simulink model "bh_3d_pend_COMPONENT_MODEL"  (R2021b)
settings: Solver=ode45  StartTime=0.0  StopTime=10.0  RelTol=1e-5
undefined symbols (not defined in the file or in its folder): g, Lx, Ly, Lz, M_cart, m_pend, q0, q0_dot
settings Model: Creator=bhorton  LastModifiedBy=bhorton
settings SolverCC: ZeroCrossAlgorithm=Adaptive  AlgebraicLoopSolver=TrustRegion
settings DataIOCC: ReturnWorkspaceOutputs=off
settings DebuggingCC: SFMachineParentedDataDiag=warning  ArithmeticOperatorsInVariantConditions=warning
settings SFSimCC: SimUseLocalCustomCode=off  CustomCodeUndefinedFunction=UseInterfaceOnly
settings RTWCC: RTWUseLocalCustomCode=off
settings CodeAppCC: StateflowObjectComments=on

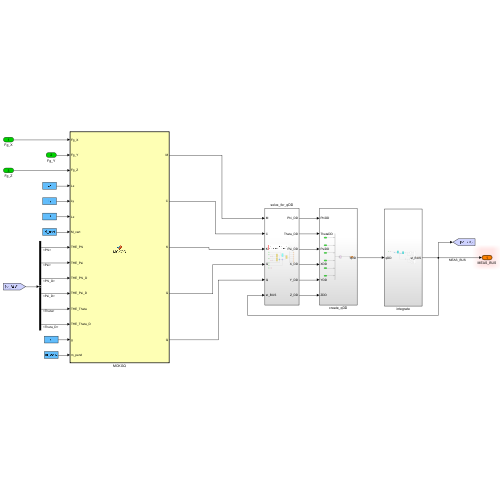
[thumbnail: Simulink's stored preview of the top-level diagram]
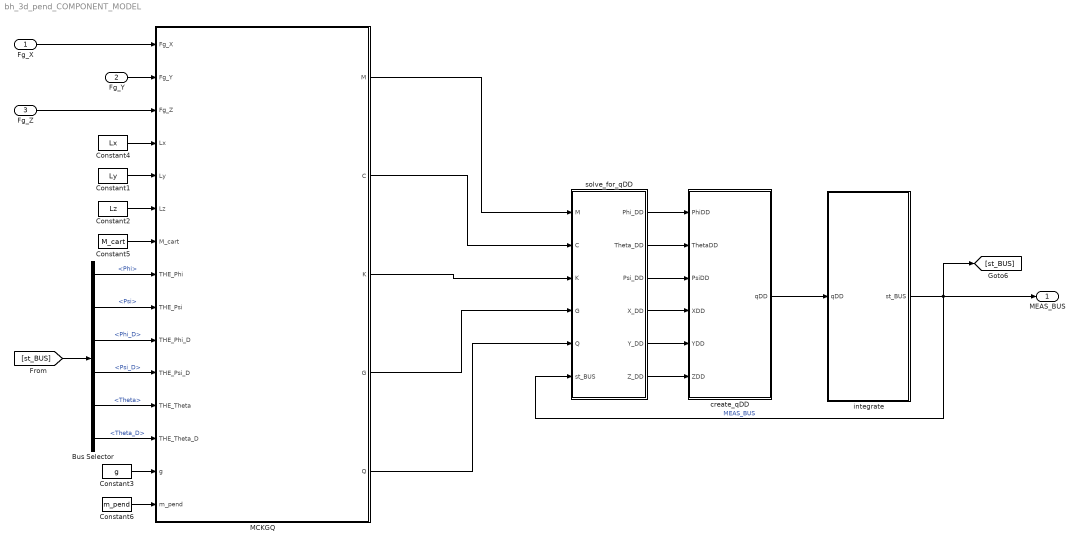
== system bh_3d_pend_COMPONENT_MODEL ==
  Fg_X : Inport
  Fg_Y : Inport  Port=2
  Fg_Z : Inport  Port=3
  Bus Selector : BusSelector  OutputSignals=Pos_list.Phi,Pos_list.Psi,Vel_list.Phi_D,Vel_list.Psi_D,Pos_list.Theta,Vel_list.Theta_D
  Constant1 : Constant  Value=Ly  OutDataTypeStr=Inherit: Inherit via back propagation
  Constant2 : Constant  Value=Lz  OutDataTypeStr=Inherit: Inherit via back propagation
  Constant3 : Constant  Value=g  OutDataTypeStr=Inherit: Inherit via back propagation
  Constant4 : Constant  Value=Lx  OutDataTypeStr=Inherit: Inherit via back propagation
  Constant5 : Constant  Value=M_cart  OutDataTypeStr=Inherit: Inherit via back propagation
  Constant6 : Constant  Value=m_pend  OutDataTypeStr=Inherit: Inherit via back propagation
  MCKGQ : MATLAB Function  TreatAsAtomicUnit=on
  create_qDD : Subsystem
  integrate : Subsystem
  solve_for_qDD : Subsystem
  MEAS_BUS : Outport  OutDataTypeStr=Bus: MEAS_BUS_SL_3D_PEND  VectorParamsAs1DForOutWhenUnconnected=off
  wires:
  solve_for_qDD/5(Y_DD) -> create_qDD/5(YDD)
  solve_for_qDD/3(Psi_DD) -> create_qDD/3(PsiDD)
  solve_for_qDD/2(Theta_DD) -> create_qDD/2(ThetaDD)
  integrate/1(st_BUS) -> MEAS_BUS/1, solve_for_qDD/6(st_BUS), [st_BUS]  "MEAS_BUS"
  solve_for_qDD/1(Phi_DD) -> create_qDD/1(PhiDD)
  solve_for_qDD/4(X_DD) -> create_qDD/4(XDD)
  solve_for_qDD/6(Z_DD) -> create_qDD/6(ZDD)
  MCKGQ/1(M) -> solve_for_qDD/1(M)
  MCKGQ/2(C) -> solve_for_qDD/2(C)
  MCKGQ/3(K) -> solve_for_qDD/3(K)
  MCKGQ/4(G) -> solve_for_qDD/4(G)
  MCKGQ/5(Q) -> solve_for_qDD/5(Q)
  create_qDD/1(qDD) -> integrate/1(qDD)
  Fg_Y/1 -> MCKGQ/2(Fg_Y)
  Fg_X/1 -> MCKGQ/1(Fg_X)
  Fg_Z/1 -> MCKGQ/3(Fg_Z)
  Constant5/1 -> MCKGQ/7(M_cart)
  Constant2/1 -> MCKGQ/6(Lz)
  Constant1/1 -> MCKGQ/5(Ly)
  Constant4/1 -> MCKGQ/4(Lx)
  Constant3/1 -> MCKGQ/14(g)
  Constant6/1 -> MCKGQ/15(m_pend)
  [st_BUS] -> Bus Selector/1
  Bus Selector/1 -> MCKGQ/8(THE_Phi)  "<Phi>"
  Bus Selector/2 -> MCKGQ/9(THE_Psi)  "<Psi>"
  Bus Selector/6 -> MCKGQ/13(THE_Theta_D)  "<Theta_D>"
  Bus Selector/5 -> MCKGQ/12(THE_Theta)  "<Theta>"
  Bus Selector/4 -> MCKGQ/11(THE_Psi_D)  "<Psi_D>"
  Bus Selector/3 -> MCKGQ/10(THE_Phi_D)  "<Phi_D>"

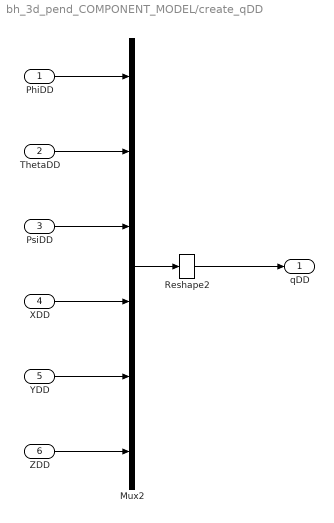
== system bh_3d_pend_COMPONENT_MODEL/create_qDD ==
  PhiDD : Inport
  ThetaDD : Inport  Port=2
  PsiDD : Inport  Port=3
  XDD : Inport  Port=4
  YDD : Inport  Port=5
  ZDD : Inport  Port=6
  Mux2 : Mux  Inputs=6
  Reshape2 : Reshape  OutputDimensionality=Column vector (2-D)
  qDD : Outport  VectorParamsAs1DForOutWhenUnconnected=off
  wires:
  PhiDD/1 -> Mux2/1
  ThetaDD/1 -> Mux2/2
  PsiDD/1 -> Mux2/3
  XDD/1 -> Mux2/4
  YDD/1 -> Mux2/5
  ZDD/1 -> Mux2/6
  Reshape2/1 -> qDD/1
  Mux2/1 -> Reshape2/1

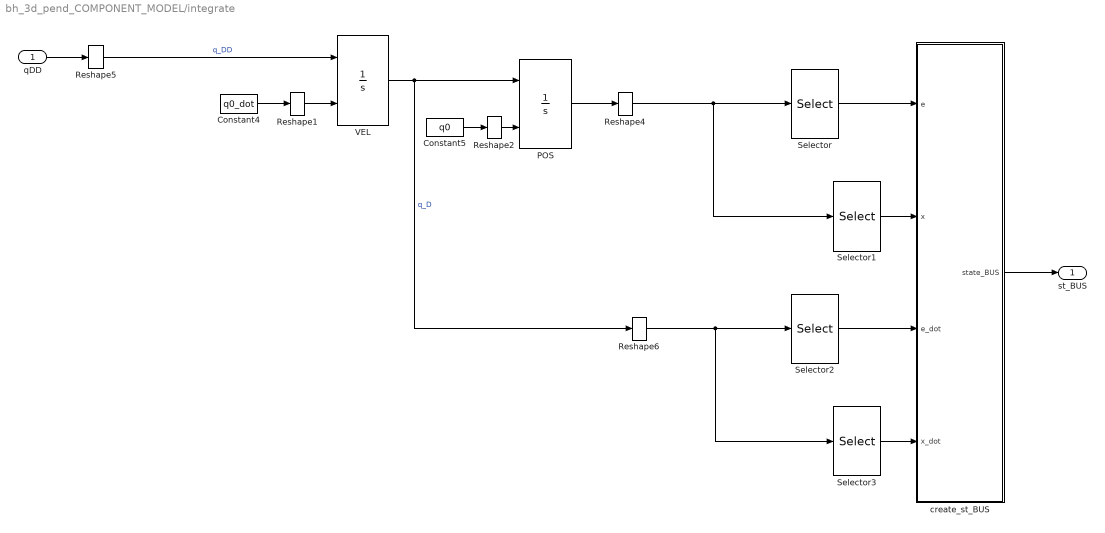
== system bh_3d_pend_COMPONENT_MODEL/integrate ==
  qDD : Inport
  Constant4 : Constant  Value=q0_dot  OutDataTypeStr=Inherit: Inherit via back propagation
  Constant5 : Constant  Value=q0  OutDataTypeStr=Inherit: Inherit via back propagation
  POS : Integrator  InitialConditionSource=external  ContinuousStateAttributes={'Phi', 'Theta', 'Psi', 'X','Y','Z'}
      settings: AttributesFormatString=%<ContinuousStateAttributes>
  Reshape{1..2,4..6} (5 alike) : Reshape  OutputDimensionality=Column vector (2-D)
  Selector : Selector  InputPortWidth=6  IndexOptions=Index vector (dialog)  Indices=1:3  OutputSizes=1
  Selector1 : Selector  InputPortWidth=6  IndexOptions=Index vector (dialog)  Indices=4:6  OutputSizes=1
  Selector2 : Selector  InputPortWidth=6  IndexOptions=Index vector (dialog)  Indices=1:3  OutputSizes=1
  Selector3 : Selector  InputPortWidth=6  IndexOptions=Index vector (dialog)  Indices=4:6  OutputSizes=1
  VEL : Integrator  InitialConditionSource=external  ContinuousStateAttributes={'Phi_D', 'Theta_D', 'Psi_D', 'X_D','Y_D','Z_D'}
      settings: AttributesFormatString=%<ContinuousStateAttributes>
  create_st_BUS : Subsystem
  st_BUS : Outport  VectorParamsAs1DForOutWhenUnconnected=off
  wires:
  qDD/1 -> Reshape5/1
  VEL/1 -> Reshape6/1, POS/1  "q_D"
  Reshape5/1 -> VEL/1  "q_DD"
  Constant5/1 -> Reshape2/1
  Constant4/1 -> Reshape1/1
  POS/1 -> Reshape4/1
  Reshape4/1 -> Selector1/1, Selector/1
  create_st_BUS/1(state_BUS) -> st_BUS/1
  Reshape1/1 -> VEL/2
  Reshape2/1 -> POS/2
  Selector3/1 -> create_st_BUS/4(x_dot)
  Selector2/1 -> create_st_BUS/3(e_dot)
  Selector1/1 -> create_st_BUS/2(x)
  Selector/1 -> create_st_BUS/1(e)
  Reshape6/1 -> Selector3/1, Selector2/1

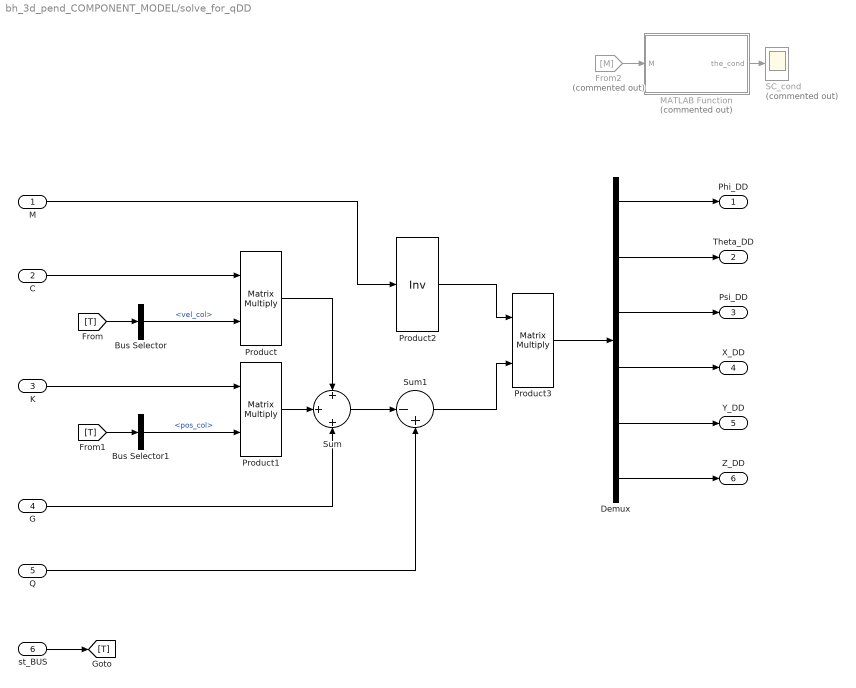
== system bh_3d_pend_COMPONENT_MODEL/solve_for_qDD ==
  M : Inport
  C : Inport  Port=2
  K : Inport  Port=3
  G : Inport  Port=4
  Q : Inport  Port=5
  st_BUS : Inport  Port=6
  Bus Selector : BusSelector  OutputSignals=vel_col
  Bus Selector1 : BusSelector  OutputSignals=pos_col
  Demux : Demux  Outputs=6
  From2 : From  Commented=on  GotoTag=M
  MATLAB Function : MATLAB Function  Commented=on  TreatAsAtomicUnit=on
  Product : Product  Multiplication=Matrix(*)
  Product1 : Product  Multiplication=Matrix(*)
  Product2 : Product  Inputs=/  Multiplication=Matrix(*)
  Product3 : Product  Multiplication=Matrix(*)
  SC_cond : Scope  Commented=on
  Sum : Sum  Inputs=+|+|+
  Sum1 : Sum  Inputs=|-+
  Phi_DD : Outport  VectorParamsAs1DForOutWhenUnconnected=off
  Theta_DD : Outport  Port=2  VectorParamsAs1DForOutWhenUnconnected=off
  Psi_DD : Outport  Port=3  VectorParamsAs1DForOutWhenUnconnected=off
  X_DD : Outport  Port=4  VectorParamsAs1DForOutWhenUnconnected=off
  Y_DD : Outport  Port=5  VectorParamsAs1DForOutWhenUnconnected=off
  Z_DD : Outport  Port=6  VectorParamsAs1DForOutWhenUnconnected=off
  wires:
  st_BUS/1 -> [T]
  C/1 -> Product/1
  [T] -> Bus Selector/1
  Bus Selector/1 -> Product/2  "<vel_col>"
  K/1 -> Product1/1
  [T] -> Bus Selector1/1
  Bus Selector1/1 -> Product1/2  "<pos_col>"
  Q/1 -> Sum1/2
  Product1/1 -> Sum/2
  G/1 -> Sum/3
  Product/1 -> Sum/1
  Sum/1 -> Sum1/1
  M/1 -> Product2/1
  Product2/1 -> Product3/1
  Sum1/1 -> Product3/2
  Product3/1 -> Demux/1
  Demux/1 -> Phi_DD/1
  Demux/2 -> Theta_DD/1
  MATLAB Function/1(the_cond) -> SC_cond/1
  Demux/3 -> Psi_DD/1
  Demux/4 -> X_DD/1
  From2/1 -> MATLAB Function/1(M)
  Demux/6 -> Z_DD/1
  Demux/5 -> Y_DD/1

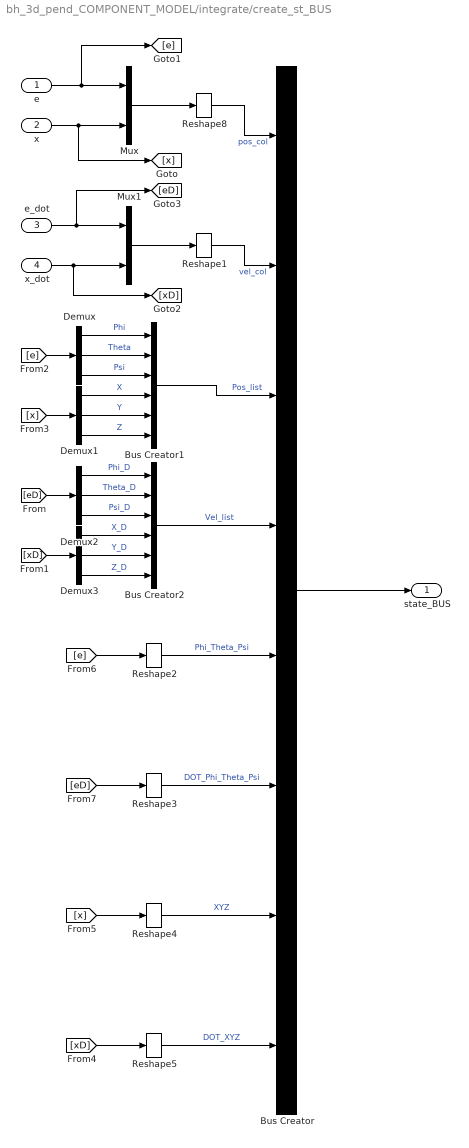
== system bh_3d_pend_COMPONENT_MODEL/integrate/create_st_BUS ==
  e : Inport
  x : Inport  Port=2
  e_dot : Inport  Port=3
  x_dot : Inport  Port=4
  Bus Creator : BusCreator  Inputs=8
  Bus Creator1 : BusCreator  Inputs=6
  Bus Creator2 : BusCreator  Inputs=6
  Demux{,1..3} (4 alike) : Demux  Outputs=3
  Mux : Mux  Inputs=2
  Mux1 : Mux  Inputs=2
  Reshape{1..5,8} (6 alike) : Reshape  OutputDimensionality=Column vector (2-D)
  state_BUS : Outport  VectorParamsAs1DForOutWhenUnconnected=off
  wires:
  e/1 -> Mux/1, [e]
  x/1 -> Mux/2, [x]
  e_dot/1 -> Mux1/1, [eD]
  x_dot/1 -> Mux1/2, [xD]
  Mux1/1 -> Reshape1/1
  Mux/1 -> Reshape8/1
  Reshape1/1 -> Bus Creator/2  "vel_col"
  Reshape8/1 -> Bus Creator/1  "pos_col"
  Bus Creator1/1 -> Bus Creator/3  "Pos_list"
  Demux/1 -> Bus Creator1/1  "Phi"
  Demux/2 -> Bus Creator1/2  "Theta"
  Demux/3 -> Bus Creator1/3  "Psi"
  Demux1/2 -> Bus Creator1/5  "Y"
  Demux1/3 -> Bus Creator1/6  "Z"
  Demux1/1 -> Bus Creator1/4  "X"
  [e] -> Demux/1
  [x] -> Demux1/1
  Bus Creator2/1 -> Bus Creator/4  "Vel_list"
  Demux2/1 -> Bus Creator2/1  "Phi_D"
  Demux2/2 -> Bus Creator2/2  "Theta_D"
  Demux2/3 -> Bus Creator2/3  "Psi_D"
  Demux3/1 -> Bus Creator2/4  "X_D"
  Demux3/2 -> Bus Creator2/5  "Y_D"
  Demux3/3 -> Bus Creator2/6  "Z_D"
  [eD] -> Demux2/1
  [xD] -> Demux3/1
  Bus Creator/1 -> state_BUS/1
  Reshape2/1 -> Bus Creator/5  "Phi_Theta_Psi"
  Reshape3/1 -> Bus Creator/6  "DOT_Phi_Theta_Psi"
  Reshape4/1 -> Bus Creator/7  "XYZ"
  Reshape5/1 -> Bus Creator/8  "DOT_XYZ"
  [xD] -> Reshape5/1
  [x] -> Reshape4/1
  [e] -> Reshape2/1
  [eD] -> Reshape3/1

== matlab function bh_3d_pend_COMPONENT_MODEL/MCKGQ ==
  data: Fg_X input; M output; Fg_Y input; Fg_Z input; Lx input; Ly input; Lz input; M_cart input; THE_Phi input; THE_Psi input; THE_Phi_D input; THE_Psi_D input; THE_Theta input; THE_Theta_D input; g input; m_pend input; C output; K output; G output; Q output
function [M,C,K,G,Q] = MCKGQ(Fg_X,Fg_Y,Fg_Z,Lx,Ly,Lz,M_cart,THE_Phi,THE_Psi,THE_Phi_D,THE_Psi_D,THE_Theta,THE_Theta_D,g,m_pend)
%#codegen

%    This function was generated by the Symbolic Math Toolbox version 9.0.
%    19-Nov-2021 15:15:08

mt1 = [(m_pend.*(-Lx.^2.*sin(THE_Theta).^2-Ly.^2.*sin(THE_Psi).^2+Lz.^2.*sin(THE_Psi).^2.*4.0+Lz.^2.*sin(THE_Theta).^2.*4.0+Lx.^2+Ly.^2+Ly.^2.*sin(THE_Psi).^2.*sin(THE_Theta).^2-Lz.^2.*sin(THE_Psi).^2.*sin(THE_Theta).^2.*4.0))./1.2e+1,m_pend.*cos(THE_Psi).*cos(THE_Theta).*sin(THE_Psi).*(Ly.^2-Lz.^2.*4.0).*(-1.0./1.2e+1),m_pend.*sin(THE_Theta).*(Ly.^2+Lz.^2.*4.0).*(-1.0./1.2e+1),(Lz.*m_pend.*(cos(THE_Phi).*sin(THE_Psi)-cos(THE_Psi).*sin(THE_Phi).*sin(THE_Theta)))./2.0,(Lz.*m_pend.*(sin(THE_Phi).*sin(THE_Psi)+cos(THE_Phi).*cos(THE_Psi).*sin(THE_Theta)))./2.0,0.0,m_pend.*cos(THE_Psi).*cos(THE_Theta).*sin(THE_Psi).*(Ly.^2-Lz.^2.*4.0).*(-1.0./1.2e+1)];
mt2 = [(m_pend.*(Ly.^2.*sin(THE_Psi).^2-Lz.^2.*sin(THE_Psi).^2.*4.0+Lx.^2+Lz.^2.*4.0))./1.2e+1,0.0,(Lz.*m_pend.*cos(THE_Phi).*cos(THE_Psi).*cos(THE_Theta))./2.0,(Lz.*m_pend.*cos(THE_Psi).*cos(THE_Theta).*sin(THE_Phi))./2.0,Lz.*m_pend.*cos(THE_Psi).*sin(THE_Theta).*(-1.0./2.0),m_pend.*sin(THE_Theta).*(Ly.^2+Lz.^2.*4.0).*(-1.0./1.2e+1),0.0,(m_pend.*(Ly.^2+Lz.^2.*4.0))./1.2e+1,(Lz.*m_pend.*(cos(THE_Psi).*sin(THE_Phi)-cos(THE_Phi).*sin(THE_Psi).*sin(THE_Theta)))./2.0,Lz.*m_pend.*(cos(THE_Phi).*cos(THE_Psi)+sin(THE_Phi).*sin(THE_Psi).*sin(THE_Theta)).*(-1.0./2.0),Lz.*m_pend.*cos(THE_Theta).*sin(THE_Psi).*(-1.0./2.0),(Lz.*m_pend.*(cos(THE_Phi).*sin(THE_Psi)-cos(THE_Psi).*sin(THE_Phi).*sin(THE_Theta)))./2.0,(Lz.*m_pend.*cos(THE_Phi).*cos(THE_Psi).*cos(THE_Theta))./2.0];
mt3 = [(Lz.*m_pend.*(cos(THE_Psi).*sin(THE_Phi)-cos(THE_Phi).*sin(THE_Psi).*sin(THE_Theta)))./2.0,M_cart+m_pend,0.0,0.0,(Lz.*m_pend.*(sin(THE_Phi).*sin(THE_Psi)+cos(THE_Phi).*cos(THE_Psi).*sin(THE_Theta)))./2.0,(Lz.*m_pend.*cos(THE_Psi).*cos(THE_Theta).*sin(THE_Phi))./2.0,Lz.*m_pend.*(cos(THE_Phi).*cos(THE_Psi)+sin(THE_Phi).*sin(THE_Psi).*sin(THE_Theta)).*(-1.0./2.0),0.0,M_cart+m_pend,0.0,0.0,Lz.*m_pend.*cos(THE_Psi).*sin(THE_Theta).*(-1.0./2.0),Lz.*m_pend.*cos(THE_Theta).*sin(THE_Psi).*(-1.0./2.0),0.0,0.0,M_cart+m_pend];
M = reshape([mt1,mt2,mt3],6,6);
if nargout > 1
    mt4 = [m_pend.*cos(THE_Theta).*(Lx.^2.*THE_Theta_D.*sin(THE_Theta)-Ly.^2.*THE_Theta_D.*sin(THE_Theta)+Ly.^2.*THE_Theta_D.*cos(THE_Psi).^2.*sin(THE_Theta)-Lz.^2.*THE_Theta_D.*cos(THE_Psi).^2.*sin(THE_Theta).*4.0+Ly.^2.*THE_Psi_D.*cos(THE_Psi).*cos(THE_Theta).*sin(THE_Psi)-Lz.^2.*THE_Psi_D.*cos(THE_Psi).*cos(THE_Theta).*sin(THE_Psi).*4.0).*(-1.0./6.0),(m_pend.*cos(THE_Theta).*(Ly.^2.*THE_Psi_D.*2.0+Lx.^2.*THE_Phi_D.*sin(THE_Theta)-Ly.^2.*THE_Phi_D.*sin(THE_Theta)-Ly.^2.*THE_Psi_D.*cos(THE_Psi).^2.*2.0+Lz.^2.*THE_Psi_D.*cos(THE_Psi).^2.*8.0+Ly.^2.*THE_Phi_D.*cos(THE_Psi).^2.*sin(THE_Theta)-Lz.^2.*THE_Phi_D.*cos(THE_Psi).^2.*sin(THE_Theta).*4.0))./1.2e+1];
    mt5 = [m_pend.*cos(THE_Theta).*(Ly.^2.*THE_Theta_D.*2.0-Ly.^2.*THE_Theta_D.*cos(THE_Psi).^2.*2.0+Lz.^2.*THE_Theta_D.*cos(THE_Psi).^2.*8.0-Ly.^2.*THE_Phi_D.*cos(THE_Psi).*cos(THE_Theta).*sin(THE_Psi)+Lz.^2.*THE_Phi_D.*cos(THE_Psi).*cos(THE_Theta).*sin(THE_Psi).*4.0).*(-1.0./1.2e+1),Lz.*m_pend.*(THE_Psi_D.*cos(THE_Phi).*cos(THE_Psi).*-2.0+THE_Phi_D.*sin(THE_Phi).*sin(THE_Psi)-THE_Psi_D.*sin(THE_Phi).*sin(THE_Psi).*sin(THE_Theta).*2.0+THE_Phi_D.*cos(THE_Phi).*cos(THE_Psi).*sin(THE_Theta)+THE_Theta_D.*cos(THE_Psi).*cos(THE_Theta).*sin(THE_Phi).*2.0).*(-1.0./2.0),(Lz.*m_pend.*(THE_Phi_D.*cos(THE_Phi).*sin(THE_Psi)+THE_Psi_D.*cos(THE_Psi).*sin(THE_Phi).*2.0+THE_Theta_D.*cos(THE_Phi).*cos(THE_Psi).*cos(THE_Theta).*2.0-THE_Phi_D.*cos(THE_Psi).*sin(THE_Phi).*sin(THE_Theta)-THE_Psi_D.*cos(THE_Phi).*sin(THE_Psi).*sin(THE_Theta).*2.0))./2.0,0.0];
    mt6 = [m_pend.*(Lz.^2.*THE_Psi_D.*cos(THE_Theta).*8.0+Ly.^2.*THE_Psi_D.*cos(THE_Psi).^2.*cos(THE_Theta).*2.0-Lz.^2.*THE_Psi_D.*cos(THE_Psi).^2.*cos(THE_Theta).*8.0-Ly.^2.*THE_Theta_D.*cos(THE_Psi).*sin(THE_Psi).*sin(THE_Theta)+Lz.^2.*THE_Theta_D.*cos(THE_Psi).*sin(THE_Psi).*sin(THE_Theta).*4.0).*(-1.0./1.2e+1),(THE_Psi_D.*m_pend.*sin(THE_Psi.*2.0).*(Ly.^2-Lz.^2.*4.0))./1.2e+1,THE_Theta_D.*m_pend.*sin(THE_Psi.*2.0).*(Ly.^2-Lz.^2.*4.0).*(-1.0./2.4e+1),Lz.*m_pend.*cos(THE_Phi).*(THE_Psi_D.*cos(THE_Theta).*sin(THE_Psi).*2.0+THE_Theta_D.*cos(THE_Psi).*sin(THE_Theta)).*(-1.0./2.0),Lz.*m_pend.*sin(THE_Phi).*(THE_Psi_D.*cos(THE_Theta).*sin(THE_Psi).*2.0+THE_Theta_D.*cos(THE_Psi).*sin(THE_Theta)).*(-1.0./2.0),Lz.*m_pend.*(THE_Theta_D.*cos(THE_Psi).*cos(THE_Theta)-THE_Psi_D.*sin(THE_Psi).*sin(THE_Theta).*2.0).*(-1.0./2.0),0.0,0.0,0.0];
    mt7 = [Lz.*THE_Psi_D.*m_pend.*(sin(THE_Phi).*sin(THE_Psi)+cos(THE_Phi).*cos(THE_Psi).*sin(THE_Theta)).*(-1.0./2.0),(Lz.*THE_Psi_D.*m_pend.*(cos(THE_Phi).*sin(THE_Psi)-cos(THE_Psi).*sin(THE_Phi).*sin(THE_Theta)))./2.0,Lz.*THE_Psi_D.*m_pend.*cos(THE_Psi).*cos(THE_Theta).*(-1.0./2.0),0.0,0.0,0.0,0.0,0.0,0.0,0.0,0.0,0.0,0.0,0.0,0.0,0.0,0.0,0.0,0.0,0.0,0.0];
    C = reshape([mt4,mt5,mt6,mt7],6,6);
end
if nargout > 2
    K = reshape([0.0,0.0,0.0,0.0,0.0,0.0,0.0,0.0,0.0,0.0,0.0,0.0,0.0,0.0,0.0,0.0,0.0,0.0,0.0,0.0,0.0,0.0,0.0,0.0,0.0,0.0,0.0,0.0,0.0,0.0,0.0,0.0,0.0,0.0,0.0,0.0],[6,6]);
end
if nargout > 3
    G = [0.0;Lz.*g.*m_pend.*cos(THE_Psi).*sin(THE_Theta).*(-1.0./2.0);Lz.*g.*m_pend.*cos(THE_Theta).*sin(THE_Psi).*(-1.0./2.0);0.0;0.0;g.*(M_cart+m_pend)];
end
if nargout > 4
    Q = [0.0;0.0;0.0;Fg_X;Fg_Y;Fg_Z];
end

== matlab function bh_3d_pend_COMPONENT_MODEL/solve_for_qDD/MATLAB Function ==
  data: M input; the_cond output
function the_cond = COND(M)
%#codegen

the_cond = cond(M);

end
